simulink library "planarBATctrllr_ul"  (R2018b)
settings: Solver=VariableStepAuto  StartTime=0.0  StopTime=10.0  RelTol=1e-3
values from neighbouring files (symbols this model uses):
  kd = 4*kp    (= 8)    [BAT_ts.m]
  kp = 2    [BAT_ts.m]
  tau = 0.5    [BAT_ts.m]
libraries: filteredPIDController_ul x1
settings Model: Creator=Ayaz  LastModifiedBy=Ayaz

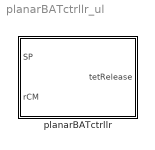
== system planarBATctrllr_ul ==
  planarBATctrllr : Subsystem  mask{kp=kp, kd=kd, tau=tau}
      mask prompts: kp "Proportional Gain, kp"; kd "Derivative Gain, kd"; tau "Time Constant, s"
      mask TypeOptions kp: filteredPIDController/kp
      mask TypeOptions kd: filteredPIDController/kd
      mask TypeOptions tau: filteredPIDController/Value

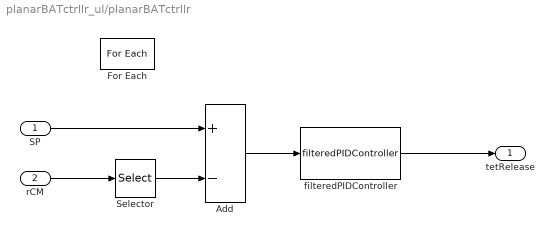
== system planarBATctrllr_ul/planarBATctrllr ==
  SP : Inport  Partition=on  PartitionDimension=2  PartitionWidth=1  PartitionOffset=0
  rCM : Inport  Port=2  Partition=on  PartitionDimension=2  PartitionWidth=1  PartitionOffset=0
  Add : Sum  Inputs=+-
  For Each : ForEach  DisableCoverage=on  IndexMode=One-based
  Selector : Selector  InputPortWidth=2  IndexOptions=Index vector (dialog)  Indices=2  OutputSizes=1
  filteredPIDController : filteredPIDController_ul/filteredPIDController  kp=kp  ki=0  kd=kd  Value=tau
  tetRelease : Outport  ConcatenationDimension=2
  wires:
  SP/1 -> Add/1
  rCM/1 -> Selector/1
  Selector/1 -> Add/2
  Add/1 -> filteredPIDController/1
  filteredPIDController/1 -> tetRelease/1
